simulink model "HIL_UDP_Test"  (R2020a)
settings: Solver=VariableStepAuto  StartTime=0.0  StopTime=10  RelTol=1e-3
undefined symbols (not defined in the file): f
libraries: instrumentlib x2, dspnetwork x2
settings Model: Creator=cihad  LastModifiedBy=waldene
settings DataIOCC: ReturnWorkspaceOutputs=off
settings DebuggingCC: ArithmeticOperatorsInVariantConditions=warning
settings SFSimCC: SimUseLocalCustomCode=off  CustomCodeUndefinedFunction=UseInterfaceOnly
settings RTWCC: RTWUseLocalCustomCode=off

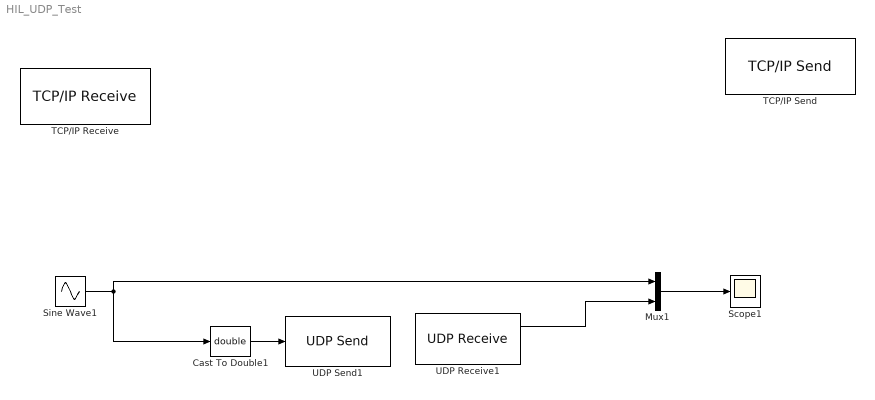
== system HIL_UDP_Test ==
  Cast To Double1 : DataTypeConversion  OutDataTypeStr=double
  Mux1 : Mux  Inputs=2
  Scope1 : Scope
  Sine Wave1 : Sin  SampleTime=0.01
  TCP/IP Receive : instrumentlib/TCP//IP Receive  Port=80  DataSize=[1 1]  EnableBlockingMode=on  Timeout=10  SampleTime=0.01  DataType=uint8  ByteOrder=BigEndian  ASCIIFormatting=%f,  Terminator=LF
  TCP/IP Send : instrumentlib/TCP//IP Send  Port=80  EnableBlockingMode=on  Timeout=10  ByteOrder=BigEndian  TransferDelay=on
  UDP Receive1 : dspnetwork/UDP Receive  localURL='0.0.0.0'  localPort=26000  remoteURL='0.0.0.0'  remotePort=-1  recvBufferSize=8192  dims=1  signalDatatype=double  isComplex=off  isVarSize=off  showBlockingTime=off  blockingTime=0  sampletime=0.001  blockPlatform=[]
  UDP Send1 : dspnetwork/UDP Send  remoteURL='127.0.0.1'  remotePort=25000  localURL='0.0.0.0'  localPortSource=Automatically determine  localPort=-1  sendBufferSize=8192  sampletime=-1  blockPlatform=[]  separateLengthPort=0
  wires:
  Mux1/1 -> Scope1/1
  Sine Wave1/1 -> Mux1/1, Cast To Double1/1
  UDP Receive1/1 -> Mux1/2
  Cast To Double1/1 -> UDP Send1/1
